simulink model "motorCC_tp2"  (R2025a)
settings: Solver=VariableStepAuto  StartTime=0.0  StopTime=3000  RelTol=1e-3
undefined symbols (not defined in the file or in its folder): dspblkCoreblockFVToolHelper, gcbh
libraries: simulink x2

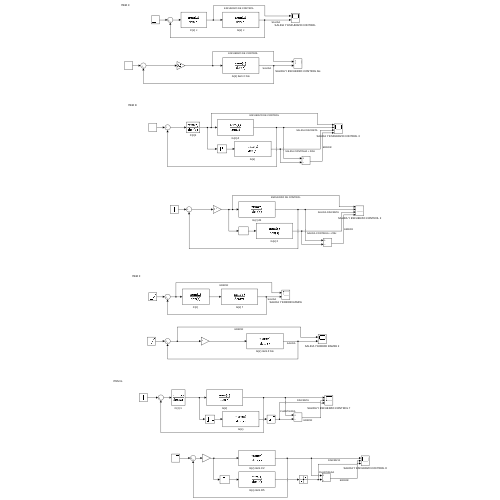
[thumbnail: Simulink's stored preview of the top-level diagram]
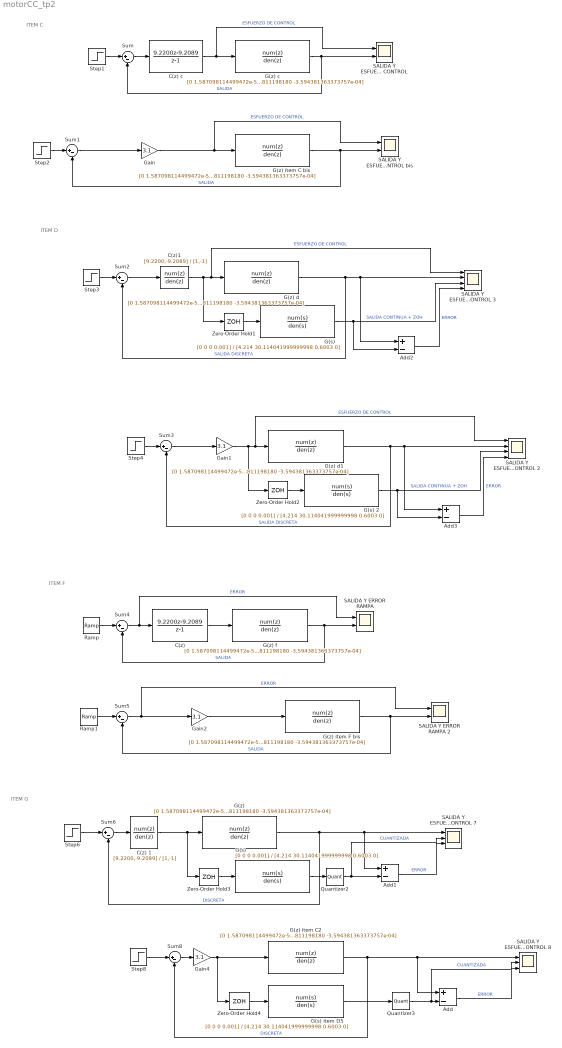
== system motorCC_tp2 ==
  note: ITEM G
  note: ITEM F
  note: ITEM C
  note: ITEM D
  Add{,1..3} (4 alike) : Sum  Inputs=+-
  "C(z) " : DiscreteTransferFcn  LoadFcn=dspblkCoreblockFVToolHelper(gcbh,'load');  Numerator=[9.2200,-9.2089]  Denominator=[1,-1]  SampleTime=1.1098
      settings: CopyFcn=dspblkCoreblockFVToolHelper(gcbh,'copy');  DeleteFcn=dspblkCoreblockFVToolHelper(gcbh,'close');  ModelCloseFcn=dspblkCoreblockFVToolHelper(gcbh,'close');  PreSaveFcn=dspblkCoreblockFVToolHelper(gcbh,'presave');  PostSaveFcn=dspblkCoreblockFVToolHelper(gcbh,'postsave');  CloseFcn=dspblkCoreblockFVToolHelper(gcbh,'close');
  C(z) 1 : DiscreteTransferFcn  LoadFcn=dspblkCoreblockFVToolHelper(gcbh,'load');  Numerator=[9.2200,-9.2089]  Denominator=[1,-1]  SampleTime=1.1098
      settings: CopyFcn=dspblkCoreblockFVToolHelper(gcbh,'copy');  DeleteFcn=dspblkCoreblockFVToolHelper(gcbh,'close');  ModelCloseFcn=dspblkCoreblockFVToolHelper(gcbh,'close');  PreSaveFcn=dspblkCoreblockFVToolHelper(gcbh,'presave');  PostSaveFcn=dspblkCoreblockFVToolHelper(gcbh,'postsave');  CloseFcn=dspblkCoreblockFVToolHelper(gcbh,'close');
  C(z) c : DiscreteTransferFcn  LoadFcn=dspblkCoreblockFVToolHelper(gcbh,'load');  Numerator=[9.2200,-9.2089]  Denominator=[1,-1]  SampleTime=1.1098
      settings: CopyFcn=dspblkCoreblockFVToolHelper(gcbh,'copy');  DeleteFcn=dspblkCoreblockFVToolHelper(gcbh,'close');  ModelCloseFcn=dspblkCoreblockFVToolHelper(gcbh,'close');  PreSaveFcn=dspblkCoreblockFVToolHelper(gcbh,'presave');  PostSaveFcn=dspblkCoreblockFVToolHelper(gcbh,'postsave');  CloseFcn=dspblkCoreblockFVToolHelper(gcbh,'close');
  C(z)1 : DiscreteTransferFcn  LoadFcn=dspblkCoreblockFVToolHelper(gcbh,'load');  Numerator=[9.2200,-9.2089]  Denominator=[1,-1]  SampleTime=1.1098
      settings: CopyFcn=dspblkCoreblockFVToolHelper(gcbh,'copy');  DeleteFcn=dspblkCoreblockFVToolHelper(gcbh,'close');  ModelCloseFcn=dspblkCoreblockFVToolHelper(gcbh,'close');  PreSaveFcn=dspblkCoreblockFVToolHelper(gcbh,'presave');  PostSaveFcn=dspblkCoreblockFVToolHelper(gcbh,'postsave');  CloseFcn=dspblkCoreblockFVToolHelper(gcbh,'close');
  G(s) : TransferFcn  Numerator=[0 0 0 0.001]  Denominator=[4.214 30.114041999999998 0.6003 0]
  "G(s) " : TransferFcn  Numerator=[0 0 0 0.001]  Denominator=[4.214 30.114041999999998 0.6003 0]
  G(s) 2 : TransferFcn  Numerator=[0 0 0 0.001]  Denominator=[4.214 30.114041999999998 0.6003 0]
  G(s) item D5 : TransferFcn  Numerator=[0 0 0 0.001]  Denominator=[4.214 30.114041999999998 0.6003 0]
  G(z) : DiscreteTransferFcn  LoadFcn=dspblkCoreblockFVToolHelper(gcbh,'load');  Numerator=[0 1.587098114499472e-5 2.404465224969516e-5 6.336036425624988e-7]  Denominator=[1 -1.978426373061843 0.978785811198180 -3.594381363373757e-04]  SampleTime=1.1098
      settings: CopyFcn=dspblkCoreblockFVToolHelper(gcbh,'copy');  DeleteFcn=dspblkCoreblockFVToolHelper(gcbh,'close');  ModelCloseFcn=dspblkCoreblockFVToolHelper(gcbh,'close');  PreSaveFcn=dspblkCoreblockFVToolHelper(gcbh,'presave');  PostSaveFcn=dspblkCoreblockFVToolHelper(gcbh,'postsave');  CloseFcn=dspblkCoreblockFVToolHelper(gcbh,'close');
  G(z) c : DiscreteTransferFcn  LoadFcn=dspblkCoreblockFVToolHelper(gcbh,'load');  Numerator=[0 1.587098114499472e-5 2.404465224969516e-5 6.336036425624988e-7]  Denominator=[1 -1.978426373061843 0.978785811198180 -3.594381363373757e-04]  SampleTime=1.1098
      settings: CopyFcn=dspblkCoreblockFVToolHelper(gcbh,'copy');  DeleteFcn=dspblkCoreblockFVToolHelper(gcbh,'close');  ModelCloseFcn=dspblkCoreblockFVToolHelper(gcbh,'close');  PreSaveFcn=dspblkCoreblockFVToolHelper(gcbh,'presave');  PostSaveFcn=dspblkCoreblockFVToolHelper(gcbh,'postsave');  CloseFcn=dspblkCoreblockFVToolHelper(gcbh,'close');
  G(z) d : DiscreteTransferFcn  LoadFcn=dspblkCoreblockFVToolHelper(gcbh,'load');  Numerator=[0 1.587098114499472e-5 2.404465224969516e-5 6.336036425624988e-7]  Denominator=[1 -1.978426373061843 0.978785811198180 -3.594381363373757e-04]  SampleTime=1.1098
      settings: CopyFcn=dspblkCoreblockFVToolHelper(gcbh,'copy');  DeleteFcn=dspblkCoreblockFVToolHelper(gcbh,'close');  ModelCloseFcn=dspblkCoreblockFVToolHelper(gcbh,'close');  PreSaveFcn=dspblkCoreblockFVToolHelper(gcbh,'presave');  PostSaveFcn=dspblkCoreblockFVToolHelper(gcbh,'postsave');  CloseFcn=dspblkCoreblockFVToolHelper(gcbh,'close');
  G(z) d1 : DiscreteTransferFcn  LoadFcn=dspblkCoreblockFVToolHelper(gcbh,'load');  Numerator=[0 1.587098114499472e-5 2.404465224969516e-5 6.336036425624988e-7]  Denominator=[1 -1.978426373061843 0.978785811198180 -3.594381363373757e-04]  SampleTime=1.1098
      settings: CopyFcn=dspblkCoreblockFVToolHelper(gcbh,'copy');  DeleteFcn=dspblkCoreblockFVToolHelper(gcbh,'close');  ModelCloseFcn=dspblkCoreblockFVToolHelper(gcbh,'close');  PreSaveFcn=dspblkCoreblockFVToolHelper(gcbh,'presave');  PostSaveFcn=dspblkCoreblockFVToolHelper(gcbh,'postsave');  CloseFcn=dspblkCoreblockFVToolHelper(gcbh,'close');
  G(z) f : DiscreteTransferFcn  LoadFcn=dspblkCoreblockFVToolHelper(gcbh,'load');  Numerator=[0 1.587098114499472e-5 2.404465224969516e-5 6.336036425624988e-7]  Denominator=[1 -1.978426373061843 0.978785811198180 -3.594381363373757e-04]  SampleTime=1.1098
      settings: CopyFcn=dspblkCoreblockFVToolHelper(gcbh,'copy');  DeleteFcn=dspblkCoreblockFVToolHelper(gcbh,'close');  ModelCloseFcn=dspblkCoreblockFVToolHelper(gcbh,'close');  PreSaveFcn=dspblkCoreblockFVToolHelper(gcbh,'presave');  PostSaveFcn=dspblkCoreblockFVToolHelper(gcbh,'postsave');  CloseFcn=dspblkCoreblockFVToolHelper(gcbh,'close');
  G(z) item C bis : DiscreteTransferFcn  LoadFcn=dspblkCoreblockFVToolHelper(gcbh,'load');  Numerator=[0 1.587098114499472e-5 2.404465224969516e-5 6.336036425624988e-7]  Denominator=[1 -1.978426373061843 0.978785811198180 -3.594381363373757e-04]  SampleTime=1.1098
      settings: CopyFcn=dspblkCoreblockFVToolHelper(gcbh,'copy');  DeleteFcn=dspblkCoreblockFVToolHelper(gcbh,'close');  ModelCloseFcn=dspblkCoreblockFVToolHelper(gcbh,'close');  PreSaveFcn=dspblkCoreblockFVToolHelper(gcbh,'presave');  PostSaveFcn=dspblkCoreblockFVToolHelper(gcbh,'postsave');  CloseFcn=dspblkCoreblockFVToolHelper(gcbh,'close');
  G(z) item C2 : DiscreteTransferFcn  LoadFcn=dspblkCoreblockFVToolHelper(gcbh,'load');  Numerator=[0 1.587098114499472e-5 2.404465224969516e-5 6.336036425624988e-7]  Denominator=[1 -1.978426373061843 0.978785811198180 -3.594381363373757e-04]  SampleTime=1.1098
      settings: CopyFcn=dspblkCoreblockFVToolHelper(gcbh,'copy');  DeleteFcn=dspblkCoreblockFVToolHelper(gcbh,'close');  ModelCloseFcn=dspblkCoreblockFVToolHelper(gcbh,'close');  PreSaveFcn=dspblkCoreblockFVToolHelper(gcbh,'presave');  PostSaveFcn=dspblkCoreblockFVToolHelper(gcbh,'postsave');  CloseFcn=dspblkCoreblockFVToolHelper(gcbh,'close');
  G(z) item F bis : DiscreteTransferFcn  LoadFcn=dspblkCoreblockFVToolHelper(gcbh,'load');  Numerator=[0 1.587098114499472e-5 2.404465224969516e-5 6.336036425624988e-7]  Denominator=[1 -1.978426373061843 0.978785811198180 -3.594381363373757e-04]  SampleTime=1.1098
      settings: CopyFcn=dspblkCoreblockFVToolHelper(gcbh,'copy');  DeleteFcn=dspblkCoreblockFVToolHelper(gcbh,'close');  ModelCloseFcn=dspblkCoreblockFVToolHelper(gcbh,'close');  PreSaveFcn=dspblkCoreblockFVToolHelper(gcbh,'presave');  PostSaveFcn=dspblkCoreblockFVToolHelper(gcbh,'postsave');  CloseFcn=dspblkCoreblockFVToolHelper(gcbh,'close');
  Gain{,1..2,4} (4 alike) : Gain  Gain=3.1
  Quantizer2 : Quantizer  QuantizationInterval=0.001367
  Quantizer3 : Quantizer  QuantizationInterval=0.001367
  Ramp : simulink/Sources/Ramp  slope=1  start=0  InitialOutput=0
  Ramp1 : simulink/Sources/Ramp  slope=1  start=0  InitialOutput=0
  SALIDA Y ERROR RAMPA : Scope  NumInputPorts=2
      settings: ActiveDisplayYMinimum=-374.70704663899016  ActiveDisplayYMaximum=3372.3634197509118  DataLoggingVariableName=ScopeData5
  SALIDA Y ERROR RAMPA 2 : Scope  NumInputPorts=2
      settings: ActiveDisplayYMinimum=-350.76841902572289  ActiveDisplayYMaximum=3156.9157712315064  DataLoggingVariableName=ScopeData6
  SALIDA Y ESFUERZO CONTROL : Scope  NumInputPorts=2
      settings: ActiveDisplayYMinimum=-2.5143806568583278  ActiveDisplayYMaximum=10.545112578402811
  SALIDA Y ESFUERZO CONTROL 2 : Scope  NumInputPorts=4
      settings: ActiveDisplayYMinimum=-0.39111785875870564  ActiveDisplayYMaximum=3.4879019843065233  DataLoggingVariableName=ScopeData4
  SALIDA Y ESFUERZO CONTROL 3 : Scope  NumInputPorts=4
      settings: ActiveDisplayYMinimum=-0.39111785875870564  ActiveDisplayYMaximum=3.4879019843065233  DataLoggingVariableName=ScopeData2
  SALIDA Y ESFUERZO CONTROL 7 : Scope  NumInputPorts=3
      settings: ActiveDisplayYMinimum=-0.12985637874544353  ActiveDisplayYMaximum=1.126255153193938  DataLoggingVariableName=ScopeData8
  SALIDA Y ESFUERZO CONTROL 8 : Scope  NumInputPorts=3
      settings: ActiveDisplayYMinimum=-0.038852792247410672  ActiveDisplayYMaximum=0.048745252043101317  DataLoggingVariableName=ScopeData9
  SALIDA Y ESFUERZO CONTROL bis : Scope  NumInputPorts=2
      settings: ActiveDisplayYMinimum=-0.38750061576955674  ActiveDisplayYMaximum=3.4875000684188397
  Step{1..4,6,8} (6 alike) : Step  Time=0  SampleTime=0
  Sum{,1..6,8} (8 alike) : Sum  Inputs=|+-
  Zero-Order Hold{1..4} (4 alike) : ZeroOrderHold  SampleTime=1.1098
  wires:
  Sum/1 -> C(z) c/1
  C(z) c/1 -> G(z) c/1, SALIDA Y ESFUERZO CONTROL/1  "ESFUERZO DE CONTROL"
  G(z) c/1 -> SALIDA Y ESFUERZO CONTROL/2, Sum/2  "SALIDA"
  Step1/1 -> Sum/1
  Step2/1 -> Sum1/1
  Gain/1 -> SALIDA Y ESFUERZO CONTROL bis/1, G(z) item C bis/1  "ESFUERZO DE CONTROL"
  Sum1/1 -> Gain/1
  G(z) item C bis/1 -> SALIDA Y ESFUERZO CONTROL bis/2, Sum1/2  "SALIDA"
  Step3/1 -> Sum2/1
  C(z)1/1 -> G(z) d/1, SALIDA Y ESFUERZO CONTROL 3/1, Zero-Order Hold1/1  "ESFUERZO DE CONTROL"
  G(z) d/1 -> Add2/1, SALIDA Y ESFUERZO CONTROL 3/2, Sum2/2  "SALIDA DISCRETA"
  Zero-Order Hold1/1 -> "G(s) "/1
  "G(s) "/1 -> Add2/2, SALIDA Y ESFUERZO CONTROL 3/3  "SALIDA CONTINUA + ZOH"
  Ramp/1 -> Sum4/1
  "C(z) "/1 -> G(z) f/1
  Sum4/1 -> SALIDA Y ERROR RAMPA/1, "C(z) "/1  "ERROR"
  G(z) f/1 -> SALIDA Y ERROR RAMPA/2, Sum4/2  "SALIDA"
  Ramp1/1 -> Sum5/1
  G(z) item F bis/1 -> SALIDA Y ERROR RAMPA 2/2, Sum5/2  "SALIDA"
  Gain2/1 -> G(z) item F bis/1
  Sum5/1 -> SALIDA Y ERROR RAMPA 2/1, Gain2/1  "ERROR"
  C(z) 1/1 -> G(z)/1, Zero-Order Hold3/1
  Step6/1 -> Sum6/1
  G(z)/1 -> SALIDA Y ESFUERZO CONTROL 7/1, Add1/1, Sum6/2  "DISCRETA"
  Zero-Order Hold3/1 -> G(s)/1
  G(s)/1 -> Quantizer2/1
  Quantizer2/1 -> Add1/2, SALIDA Y ESFUERZO CONTROL 7/2  "CUANTIZADA"
  Quantizer3/1 -> Add/2, SALIDA Y ESFUERZO CONTROL 8/2  "CUANTIZADA"
  Zero-Order Hold4/1 -> G(s) item D5/1
  Step8/1 -> Sum8/1
  G(s) item D5/1 -> Quantizer3/1
  Gain4/1 -> Zero-Order Hold4/1, G(z) item C2/1
  Sum8/1 -> Gain4/1
  G(z) item C2/1 -> SALIDA Y ESFUERZO CONTROL 8/1, Add/1, Sum8/2  "DISCRETA"
  Add/1 -> SALIDA Y ESFUERZO CONTROL 8/3  "ERROR"
  Add1/1 -> SALIDA Y ESFUERZO CONTROL 7/3  "ERROR"
  Add2/1 -> SALIDA Y ESFUERZO CONTROL 3/4  "ERROR"
  Sum2/1 -> C(z)1/1
  Zero-Order Hold2/1 -> G(s) 2/1
  G(z) d1/1 -> Add3/1, SALIDA Y ESFUERZO CONTROL 2/2, Sum3/2  "SALIDA DISCRETA"
  Step4/1 -> Sum3/1
  Gain1/1 -> G(z) d1/1, SALIDA Y ESFUERZO CONTROL 2/1, Zero-Order Hold2/1  "ESFUERZO DE CONTROL"
  G(s) 2/1 -> Add3/2, SALIDA Y ESFUERZO CONTROL 2/3  "SALIDA CONTINUA + ZOH"
  Add3/1 -> SALIDA Y ESFUERZO CONTROL 2/4  "ERROR"
  Sum3/1 -> Gain1/1
  Sum6/1 -> C(z) 1/1
